simulink subsystem "Position_Calculation_ThorneFleissner"  (R2020b)
settings: Solver=VariableStepAuto  StartTime=0.0  StopTime=10.0  RelTol=1e-3
settings Model: Creator=rthom  LastModifiedBy=rthom

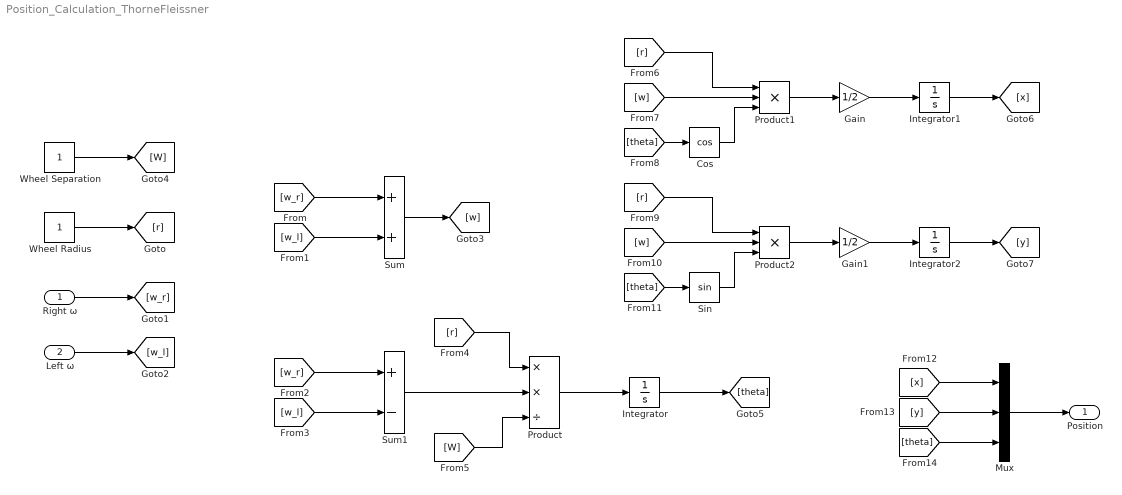
== system Position_Calculation_ThorneFleissner ==
  Right ω : Inport
  Left ω : Inport  Port=2
  Cos : Trigonometry  Operator=cos
  Gain : Gain  Gain=1/2
  Gain1 : Gain  Gain=1/2
  Integrator : Integrator
  Integrator1 : Integrator
  Integrator2 : Integrator
  Mux : Mux  Inputs=3
  Product : Product  Inputs=**/
  Product1 : Product  Inputs=3
  Product2 : Product  Inputs=3
  Sin : Trigonometry
  Sum : Sum
  Sum1 : Sum  Inputs=+-
  Wheel Radius : Constant
  Wheel Separation : Constant
  Position : Outport
  wires:
  Wheel Radius/1 -> [r]
  Right ω/1 -> [w_r]
  Left ω/1 -> [w_l]
  [w_r] -> Sum/1
  [w_l] -> Sum/2
  Sum/1 -> [w]
  [w_l] -> Sum1/2
  [w_r] -> Sum1/1
  [r] -> Product/1
  Sum1/1 -> Product/2
  Wheel Separation/1 -> [W]
  [W] -> Product/3
  Product/1 -> Integrator/1
  Integrator/1 -> [theta]
  [theta] -> Cos/1
  Cos/1 -> Product1/3
  [w] -> Product1/2
  [r] -> Product1/1
  Sin/1 -> Product2/3
  [theta] -> Sin/1
  [w] -> Product2/2
  [r] -> Product2/1
  Product1/1 -> Gain/1
  Product2/1 -> Gain1/1
  Gain1/1 -> Integrator2/1
  Gain/1 -> Integrator1/1
  Integrator2/1 -> [y]
  Integrator1/1 -> [x]
  [x] -> Mux/1
  [y] -> Mux/2
  [theta] -> Mux/3
  Mux/1 -> Position/1
